simulink model "LidarIntensityTest"  (R2026a)
settings: Solver=FixedStepDiscrete  StopTime=4
model workspace (MAT data in the model file):
  firstWarning = 1
  originalScenarioChecksum = 'D2630FF18D19558EF4F4CB681DB41729'
libraries: lidarlib x1, drivingscenarioandsensors x1
settings Model: Creator=pavanreddy  LastModifiedBy=pavanreddy

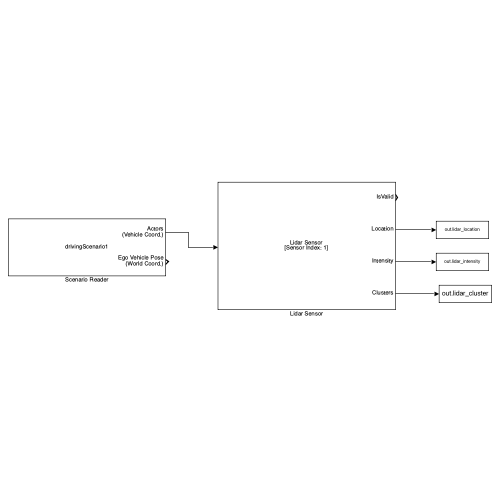
[thumbnail: Simulink's stored preview of the top-level diagram]
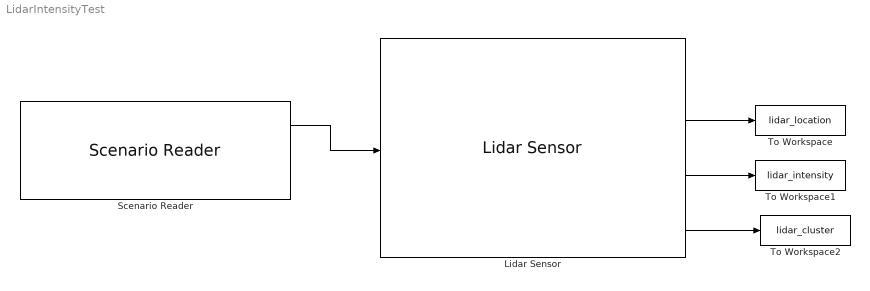
== system LidarIntensityTest ==
  Lidar Sensor : lidarlib/Lidar Sensor  SensorIndex=1  UpdateRate=0.1  Model=Custom  SensorPosition=[1.5 0 1.6]  SensorOrientation=[0 0 0]  ActorProfilesVariableName=actor_profiles  HostID=1  CoordinateSystem=Sensor  MaxRange=120  AzimuthLimits=[-180 180]  AzimuthResolution=0.16  UseCustomElevationAngles=off  ElevationAngles=[-25 -15.6 -11.3 -8.8:0.9:-4 -4:0.32:1.6 3.3 4.6 7 10.3 15]  ElevationLimits=[-20 20]  ElevationResolution=0.4  HasNoise=on  RangeAccuracy=0.01  FogVisibility=1000  Rainrate=0  HasMotionDistortion=off  FiringTimes=[]  MaterialAttributesJSON=|  EditMaterialAttributesJSON=off  OutputIntensity=on  OutputClusters=on
      | [
      | {"Material":"Aluminum","Reflectance":0.63,"Diffuseness":1,"Roughness":0.3,"Description":"Weathered aluminum metal from roof"},
      | {"Material":"Asphalt","Reflectance":0.1,"Diffuseness":1,"Roughness":0.3,"Description":"Road or construction material"},
      | {"Material":"Bark","Reflectance":0.56,"Diffuseness":1,"Roughness":0.3,"Description":"Pinus ponderosa tree bark"},
      | {"Material":"Brick","Reflectance":0.29,"Diffuseness":1,"Roughness":0.3,"Description":"Smooth-faced red building construction brick"},
      | {"Material":"Cement","Reflectance":0.35,"Diffuseness":1,"Roughness":0.3,"Description":"Cement construction concrete cinderblock"},
      | {"Material":"Concrete","Reflectance":0.33,"Diffuseness":1,"Roughness":0.3,"Description":"Road or construction material"},
      | {"Material":"Copper","Reflectance":0.57,"Diffuseness":1,"Roughness":0.3,"Description":"Weathered copper metal from roof"},
      | {"Material":"Default","Reflectance":1,"Diffuseness":1,"Roughness":0.3,"Description":"Default material attributes"},
      | {"Material":"Glass","Reflectance":0.08,"Diffuseness":1,"Roughness":0.3,"Description":"Transparent construction plate window glass"},
      | {"Material":"Grass","Reflectance":0.5,"Diffuseness":1,"Roughness":0.3,"Description":"Green Rye grass"},
      | {"Material":"Ice","Reflectance":0.017,"Diffuseness":1,"Roughness":0.3,"Description":"Ice"},
      | {"Material":"Leaves","Reflectance":0.56,"Diffuseness":1,"Roughness":0.3,"Description":"Quercus species (Oak tree) leaves"},
      | {"Material":"Marble","Reflectance":0.84,"Diffuseness":1,"Roughness":0.3,"Description":"White weathered construction marble"},
      | {"Material":"Rubber","Reflectance":0.6,"Diffuseness":1,"Roughness":0.3,"Description":"White rubberized coating from building roof"},
      | {"Material":"Snow","Reflectance":0.71,"Diffuseness":1,"Roughness":0.3,"Description":"Coarse granular snow"},
      | {"Material":"Steel","Reflectance":0.064,"Diffuseness":1,"Roughness":0.3,"Description":"Weathered, galvanized steel metal from roof"},
      | {"Material":"Tar","Reflectance":0.07,"Diffuseness":1,"Roughness":0.3,"Description":"Black, glossy construction tar"},
      | {"Material":"Terracotta","Reflectance":0.17,"Diffuseness":1,"Roughness":0.3,"Description":"Weathered terra cotta roofing tile of ceramic composite construction"},
      | {"Material":"Water","Reflectance":0.025,"Diffuseness":1,"Roughness":0.3,"Description":"Tap water"},
      | {"Material":"Wood","Reflectance":0.85,"Diffuseness":1,"Roughness":0.3,"Description":"Bare pine wood construction lumber"}
      | ]
  Scenario Reader : drivingscenarioandsensors/Scenario Reader  Priority=-1  ScenarioSource=From file  ScenarioFileName=/Users/pavanreddy/Documents/MATLAB/LidarAnalysis/drivingScenario1.mat  ScenarioVariableName=scenario  OutputCoordinateSystem=Vehicle coordinates  EgoVehicleSource=Scenario  EgoVehicleActorID=1  OrientVehiclesOnRoad=off  OutputEgoVehiclePose=on  OutputEgoVehicleState=off  SampleTime=0.1  LaneBoundaryOutput=None  LaneBoundaryDistance=0:0.5:9.5  LaneBoundaryLocation=Center of lane markings  BusNameSource=Auto  BusName=BusActors  BusNumActorsSource=Scenario  BusNumActors=100  BusName2Source=Auto  BusName2=BusLaneBoundaries  BusNumLaneBoundariesSource=Scenario  BusNumLaneBoundaries=10  BusName3Source=Auto  BusName3=BusEgoActor  BusName4Source=Auto  BusName4=BusEgoState  ShowCoordinateLabels=on  SimulateUsing=Interpreted execution
  To Workspace : ToWorkspace  VariableName=lidar_location  SaveFormat=Timeseries  SampleTime=-1
  To Workspace1 : ToWorkspace  VariableName=lidar_intensity  SaveFormat=Timeseries  SampleTime=-1
  To Workspace2 : ToWorkspace  VariableName=lidar_cluster  SaveFormat=Timeseries  SampleTime=-1
  wires:
  Lidar Sensor/2 -> To Workspace/1
  Lidar Sensor/3 -> To Workspace1/1
  Lidar Sensor/4 -> To Workspace2/1
  Scenario Reader/1 -> Lidar Sensor/1
